simulink model "model_matematyczny_regulator_2018b"  (R2018b)
settings: Solver=VariableStepAuto  StartTime=0.0  StopTime=30  RelTol=1e-3
settings Model: Creator=Admin  LastModifiedBy=Student
settings DataIOCC: ExternalInput=getinputstruct(op_trim2)  InitialState=getstatestruct(op_trim2)  ReturnWorkspaceOutputs=on
settings DebuggingCC: UnconnectedInputMsg=none  UnconnectedOutputMsg=none  UnconnectedLineMsg=none  SFMachineParentedDataDiag=error

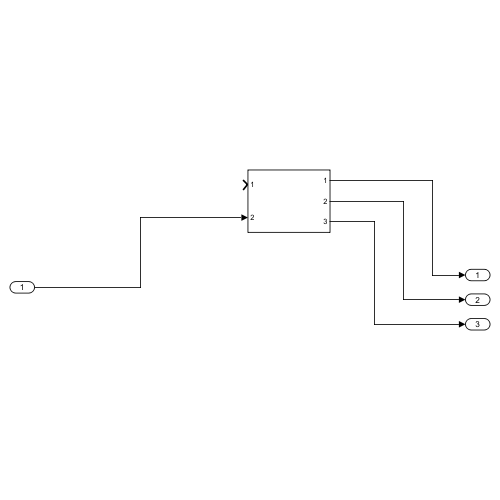
[thumbnail: Simulink's stored preview of the top-level diagram]
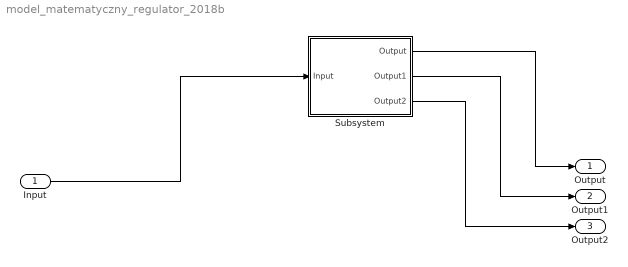
== system model_matematyczny_regulator_2018b ==
  Input : Inport
  Subsystem : Subsystem
  Output : Outport  VectorParamsAs1DForOutWhenUnconnected=on
  Output1 : Outport  Port=2  VectorParamsAs1DForOutWhenUnconnected=on
  Output2 : Outport  Port=3  VectorParamsAs1DForOutWhenUnconnected=on
  wires:
  Input/1 -> Subsystem/1(Input)
  Subsystem/1(Output) -> Output/1
  Subsystem/2(Output1) -> Output1/1
  Subsystem/3(Output2) -> Output2/1

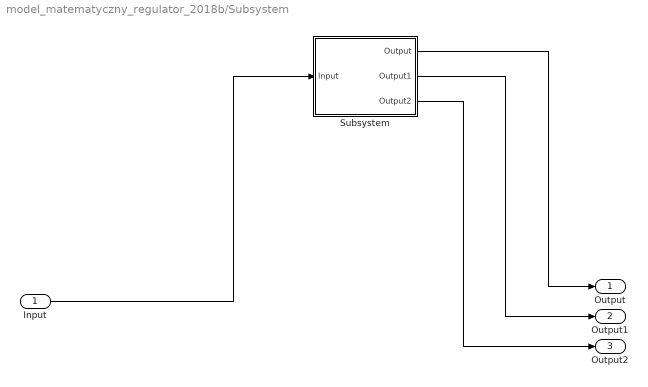
== system model_matematyczny_regulator_2018b/Subsystem ==
  Input : Inport
  Subsystem : Subsystem
  Output : Outport  VectorParamsAs1DForOutWhenUnconnected=on
  Output1 : Outport  Port=2  VectorParamsAs1DForOutWhenUnconnected=on
  Output2 : Outport  Port=3  VectorParamsAs1DForOutWhenUnconnected=on
  wires:
  Input/1 -> Subsystem/1(Input)
  Subsystem/1(Output) -> Output/1
  Subsystem/2(Output1) -> Output1/1
  Subsystem/3(Output2) -> Output2/1

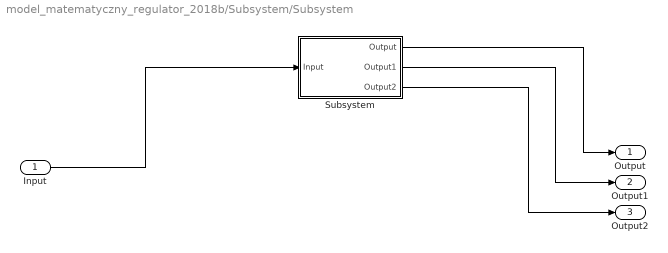
== system model_matematyczny_regulator_2018b/Subsystem/Subsystem ==
  Input : Inport
  Subsystem : Subsystem
  Output : Outport  VectorParamsAs1DForOutWhenUnconnected=on
  Output1 : Outport  Port=2  VectorParamsAs1DForOutWhenUnconnected=on
  Output2 : Outport  Port=3  VectorParamsAs1DForOutWhenUnconnected=on
  wires:
  Input/1 -> Subsystem/1(Input)
  Subsystem/1(Output) -> Output/1
  Subsystem/2(Output1) -> Output1/1
  Subsystem/3(Output2) -> Output2/1

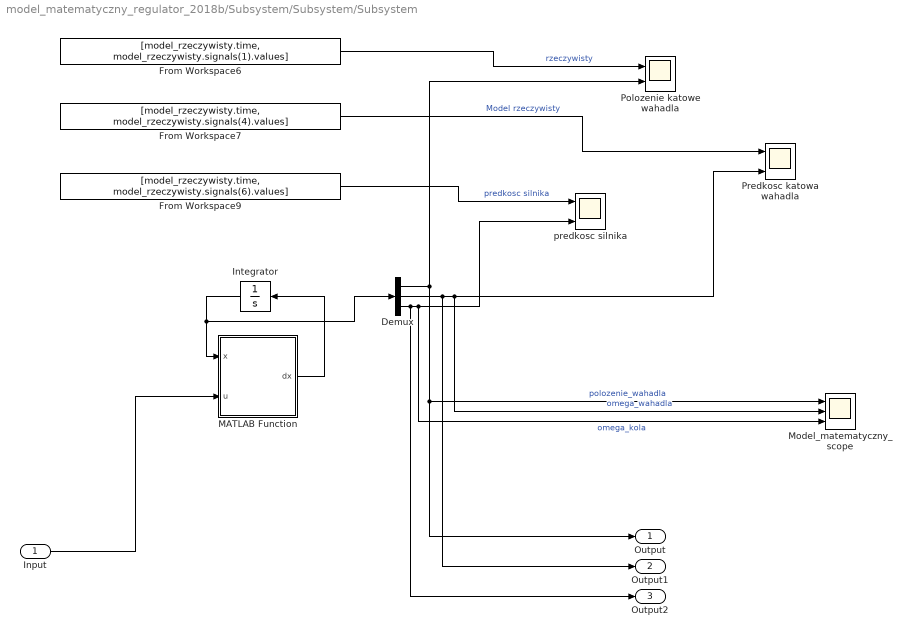
== system model_matematyczny_regulator_2018b/Subsystem/Subsystem/Subsystem ==
  Input : Inport
  Demux : Demux  Outputs=3
  From Workspace6 : FromWorkspace  VariableName=[model_rzeczywisty.time, model_rzeczywisty.signals(1).values]  SampleTime=0
  From Workspace7 : FromWorkspace  VariableName=[model_rzeczywisty.time, model_rzeczywisty.signals(4).values]  SampleTime=0
  From Workspace9 : FromWorkspace  VariableName=[model_rzeczywisty.time, model_rzeczywisty.signals(6).values]  SampleTime=0
  Integrator : Integrator  InitialCondition=[0, 0, 0]
  MATLAB Function : MATLAB Function  TreatAsAtomicUnit=on
  Model_matematyczny_scope : Scope  NumInputPorts=3
  "Polozenie katowe wahadla " : Scope  NumInputPorts=2
  "Predkosc katowa wahadla " : Scope  NumInputPorts=2
  "predkosc silnika " : Scope  NumInputPorts=2
  Output : Outport  VectorParamsAs1DForOutWhenUnconnected=on
  Output1 : Outport  Port=2  VectorParamsAs1DForOutWhenUnconnected=on
  Output2 : Outport  Port=3  VectorParamsAs1DForOutWhenUnconnected=on
  wires:
  Demux/3 -> Output2/1, Model_matematyczny_scope/3, "predkosc silnika "/2  "omega_kola"
  Demux/2 -> Output1/1, Model_matematyczny_scope/2, "Predkosc katowa wahadla "/2  "omega_wahadla"
  MATLAB Function/1(dx) -> Integrator/1
  Demux/1 -> Output/1, Model_matematyczny_scope/1, "Polozenie katowe wahadla "/2  "polozenie_wahadla"
  From Workspace7/1 -> "Predkosc katowa wahadla "/1  "Model rzeczywisty"
  Integrator/1 -> MATLAB Function/1(x), Demux/1
  From Workspace6/1 -> "Polozenie katowe wahadla "/1  "rzeczywisty"
  From Workspace9/1 -> "predkosc silnika "/1  "predkosc silnika"
  Input/1 -> MATLAB Function/2(u)

== matlab function model_matematyczny_regulator_2018b/Subsystem/Subsystem/Subsystem/MATLAB Function ==
  data: x input; u input; dx output
% function dx = fcn(x, u)
% 
% %dane wyidentyfikowane
% MgL = 0.1064;
% g = 9.81;
% kt = 0.027; % NmA
% R = 0.4; %Ohmy
% 
% mi_phi = 0.000082; 
% % mi_phi = 1.566850664740816e-04;
% % mi_theta = 0.0290; %zostało wyznaczone z drgań swobodnych 
% mi_theta = 0.0290;
% 
% G = 488.7;
% J = 0.0283; %kg*m^2
% 
% %wspołczynnik a:
% % a = 0.0023;
% % b = -0.0022;
% p = [0.002321260244060,-0.002210724041962];
% dx = [0 0 0];
% dx(1) = x(2); % pochodna polozenia
% dx(2) = (1/J)*(MgL * sin(x(1)) - mi_theta * x(2) + (((kt * kt)/R) + mi_phi) * x(3) - kt*u/R); % pochodna predkosci obrotowe belki
% dx(3) = G * (u - polyval(p, x(3))); %pochodna predkosci smigla 
% 
% end


function dx = fcn(x, u)

%dane wyidentyfikowane
MgL = 0.1264;
g = 9.81;
kt = 0.027; % NmA
ke = 0.025;
R = 2.4; %Ohmy

% mi_phi = 0.000644785835713765; 
mi_phi = 0.0000882;
% mi_theta = 0.00000132; %zostało wyznaczone z drgań swobodnych 
mi_theta = 0.0290;

G = 488.648;
% J = 0.0219; %kg*m^2
J = 0.0254;
p = [0.002314296507890,-8.816367649105842e-04];
p_volt = [11.823766233766237,0.009523809523809];
dx = [0 0 0];
dx(1) = x(2); % pochodna polozenia
% dx(2) = (1/J)*(-MgL * sin(x(1)) - mi_theta * x(2) + (((kt * ke)/R) + mi_phi) * x(3) - kt*u/R); % pochodna predkosci obrotowe belki
dx(2) = (1/J)*(-MgL * sin(x(1)) - mi_theta * x(2) - (kt * (polyval(p_volt, u) - ke * x(3)) / R) + mi_phi * x(3));
dx(3) = G * (u - polyval(p, x(3))); %pochodna predkosci smigla 

end
